simulink model "ControlBC"  (R2023b)
settings: Solver=VariableStepAuto  StartTime=0.0  StopTime=10.0  RelTol=1e-3
settings Model: Creator=USUARIO  LastModifiedBy=USUARIO

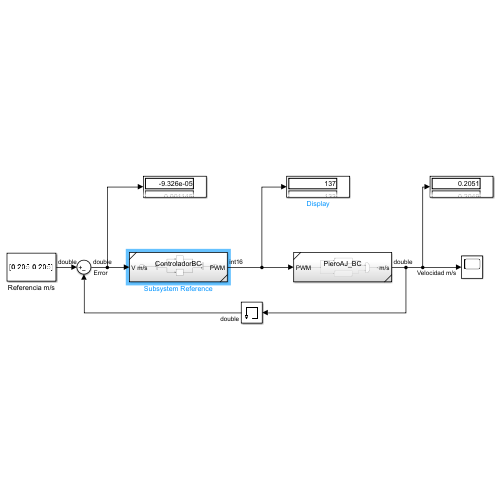
[thumbnail: Simulink's stored preview of the top-level diagram]
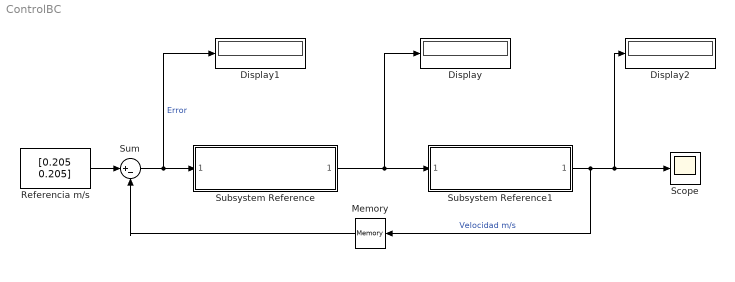
== system ControlBC ==
  Display : Display
  Display1 : Display
  Display2 : Display
  Memory : Memory
  Referencia m/s : Constant  Value=[0.205 0.205]
  Scope : Scope
  Subsystem Reference : Subsystem  ReferencedSubsystem=ControladorBC
  Subsystem Reference1 : Subsystem  ReferencedSubsystem=PieroAJ_BC
  Sum : Sum  Inputs=|+-
  wires:
  Sum/1 -> Display1/1, Subsystem Reference/1  "Error"
  Subsystem Reference/1 -> Display/1, Subsystem Reference1/1
  Referencia m/s/1 -> Sum/1
  Subsystem Reference1/1 -> Display2/1, Scope/1, Memory/1  "Velocidad m/s"
  Memory/1 -> Sum/2
